simulink model "Simple_dvig"  (R2012b)
settings: Solver=ode23tb  StartTime=0.0  StopTime=2  RelTol=1e-3
values from neighbouring files (symbols this model uses):
  f = 12    [Parameters.m]
  J = Jr + Jh    (= 0.0002754438)    [Parameters.m]
  k = 1/(3*R)    (= 0.537634408602)    [Parameters.m]
  ki = 25.5e-3*1/2    (= 0.01275)    [Parameters.m]
  kw = 30/(KV*pi)*1/2    (= 0.0127664392854)    [Parameters.m]
  R = 1.24/2    (= 0.62)    [Parameters.m]
  Te = L/R    (= 0.000451612903226)    [Parameters.m]
  Tem = 17.6e-3    (= 0.0176)    [Parameters.m]
  U = 12    [Parameters.m]
libraries: simulink x1
settings Model: Creator=botva  LastModifiedBy=botva
settings ConfigurationSet: Description=SimMechanics 2G

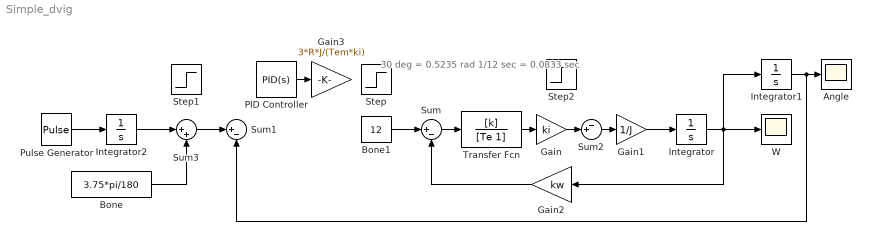
== system Simple_dvig ==
  note: 30 deg = 0.5235 rad
      | 1/12 sec = 0.0833 sec
  Angle : Scope
      settings: TimeRange=0.06  YMin=-500  YMax=500  DataFormat=Structure
  Bone : Constant  Value=3.75*pi/180
  Bone1 : Constant  Value=12
  Gain : Gain  Gain=ki
  Gain1 : Gain  Gain=1/J
  Gain2 : Gain  Gain=kw
  Gain3 : Gain  Gain=3*R*J/(Tem*ki)
  Integrator : Integrator
  Integrator1 : Integrator
  Integrator2 : Integrator
  PID Controller : simulink/Continuous/PID Controller  Controller=PID  TimeDomain=Continuous-time  SampleTime=1  IntegratorMethod=Forward Euler  FilterMethod=Forward Euler  Form=Parallel  P=115.208539177264  I=101.131824995047  D=0.0250945975978951  N=547.242728151056  InitialConditionSource=internal  InitialConditionForIntegrator=0  InitialConditionForFilter=0  ExternalReset=none  LimitOutput=off  UpperSaturationLimit=inf  LowerSaturationLimit=-inf  LinearizeAsGain=on  AntiWindupMode=none  Kb=1  TrackingMode=off  Kt=1  PParamMin=[]  PParamMax=[]  IParamMin=[]  IParamMax=[]  DParamMin=[]  DParamMax=[]  NParamMin=[]  NParamMax=[]  KbParamMin=[]  KbParamMax=[]  KtParamMin=[]  KtParamMax=[]  POutMin=[]  POutMax=[]  IOutMin=[]  IOutMax=[]  DOutMin=[]  DOutMax=[]  NOutMin=[]  NOutMax=[]  KbOutMin=[]  KbOutMax=[]  KtOutMin=[]  KtOutMax=[]  IntegratorOutMin=[]  IntegratorOutMax=[]  FilterOutMin=[]  FilterOutMax=[]  SumOutMin=[]  SumOutMax=[]  SumI1OutMin=[]  SumI1OutMax=[]  SumI2OutMin=[]  SumI2OutMax=[]  SumI3OutMin=[]  SumI3OutMax=[]  SumDOutMin=[]  SumDOutMax=[]  SaturationOutMin=[]  SaturationOutMax=[]  IntegratorContinuousStateAttributes=''  IntegratorStateMustResolveToSignalObject=off  IntegratorRTWStateStorageClass=Auto  FilterContinuousStateAttributes=''  FilterStateMustResolveToSignalObject=off  FilterRTWStateStorageClass=Auto
  Pulse Generator : DiscretePulseGenerator  PulseType=Time based  Amplitude=100*50*f*pi/6  Period=0.4  PulseWidth=0.01
  Step : Step  Time=0  After=U  SampleTime=0
  Step1 : Step  Time=0  After=pi/6+3.75*pi/180  SampleTime=0
  Step2 : Step  Time=0  After=0.0549  SampleTime=0
  Sum : Sum  Inputs=|+-
  Sum1 : Sum  Inputs=|+-
  Sum2 : Sum  Inputs=-+|
  Sum3 : Sum  Inputs=|++
  Transfer Fcn : TransferFcn  Numerator=[k]  Denominator=[Te 1]
  W : Scope
      settings: TimeRange=0.06  YMin=-500  YMax=500  SaveName=ScopeData2  DataFormat=Structure
  wires:
  Gain2/1 -> Sum/2
  Transfer Fcn/1 -> Gain/1
  Gain1/1 -> Integrator/1
  Integrator/1 -> W/1, Gain2/1, Integrator1/1
  Pulse Generator/1 -> Integrator2/1
  PID Controller/1 -> Gain3/1
  Integrator1/1 -> Angle/1, Sum1/2
  Sum/1 -> Transfer Fcn/1
  Bone1/1 -> Sum/1
  Gain/1 -> Sum2/2
  Sum2/1 -> Gain1/1
  ? -> Sum2/1
  Integrator2/1 -> Sum3/1
  Bone/1 -> Sum3/2
  Sum3/1 -> Sum1/1
